simulink model "ENEL441LabFall2012_WithNums"  (R2012b)
settings: Solver=ode45  StartTime=0.0  StopTime=10.0  RelTol=1e-3
undefined symbols (not defined in the file or in its folder): Kd, Ki, Kp
settings Model: Creator=kyle  LastModifiedBy=kyle

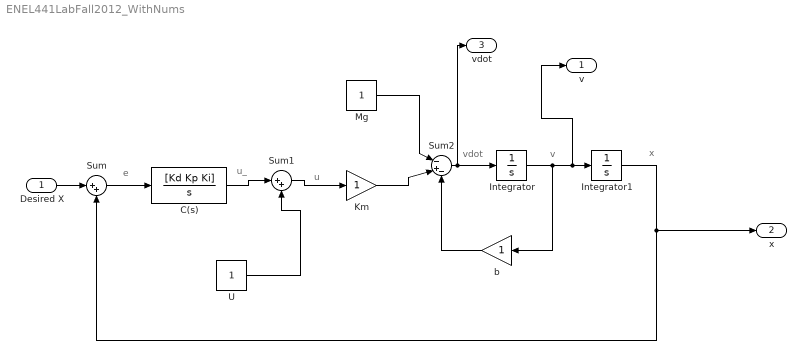
== system ENEL441LabFall2012_WithNums ==
  note: u_
  note: e
  note: u
  note: vdot
  note: v
  note: x
  Desired X : Inport
  C(s) : TransferFcn  Numerator=[Kd Kp Ki]  Denominator=[1 0]
  Integrator : Integrator
  Integrator1 : Integrator
  Km : Gain
  Mg : Constant
  Sum : Sum  Inputs=|++
  Sum1 : Sum  Inputs=|++
  Sum2 : Sum  Inputs=|-+-
  U : Constant
  b : Gain
  v : Outport
  x : Outport  Port=2
  vdot : Outport  Port=3
  wires:
  Sum/1 -> C(s)/1
  U/1 -> Sum1/2
  C(s)/1 -> Sum1/1
  Sum1/1 -> Km/1
  Km/1 -> Sum2/2
  Mg/1 -> Sum2/1
  b/1 -> Sum2/3
  Sum2/1 -> vdot/1, Integrator/1
  Integrator/1 -> b/1, v/1, Integrator1/1
  Integrator1/1 -> x/1, Sum/2
  Desired X/1 -> Sum/1
